simulink model "multiPhaseAFPM"  (R2022a)
settings: Solver=FixedStepAuto  StartTime=0.0  StopTime=T_end  FixedStep=T_sim  RelTol=1e-3
values from neighbouring files (symbols this model uses):
  fe = 0    [initializationScript.m]
  Id3_ref1 = 0    [initializationScript.m]
  Id3_ref2 = 0    [initializationScript.m]
  Id3_step = 0    [initializationScript.m]
  Id5_ref1 = 0    [initializationScript.m]
  Id5_ref2 = 0    [initializationScript.m]
  Id5_step = 0.0    (= 0)    [initializationScript.m]
  Id_ref1 = 0    [initializationScript.m]
  Id_ref2 = 0    [initializationScript.m]
  Id_step = 0    [initializationScript.m]
  Iq3_ref1 = 0    [initializationScript.m]
  Iq3_ref2 = 140    [initializationScript.m]
  Iq3_step = 0    [initializationScript.m]
  Iq5_ref1 = 0    [initializationScript.m]
  Iq5_ref2 = 0    [initializationScript.m]
  Iq5_step = 0    [initializationScript.m]
  Iq_ref1 = 0    [initializationScript.m]
  Iq_ref2 = 0    [initializationScript.m]
  Iq_step = 0    [initializationScript.m]
  L_ind1 = L1    (= 5e-05)    [initializationScript.m]
  L_ind2 = L1    (= 5e-05)    [initializationScript.m]
  L_ind3 = L1    (= 5e-05)    [initializationScript.m]
  L_ind4 = L1    (= 5e-05)    [initializationScript.m]
  L_ind5 = L1    (= 5e-05)    [initializationScript.m]
  L_ind6 = L1    (= 5e-05)    [initializationScript.m]
  L_ind7 = L1    (= 5e-05)    [initializationScript.m]
  PWM_INVERTER = 1    [initializationScript.m]
  R1 = R    (= 0.024)    [initializationScript.m]
  R2 = R    (= 0.024)    [initializationScript.m]
  R3 = R    (= 0.024)    [initializationScript.m]
  R4 = R    (= 0.024)    [initializationScript.m]
  R5 = R    (= 0.024)    [initializationScript.m]
  R6 = R    (= 0.024)    [initializationScript.m]
  R7 = R    (= 0.024)    [initializationScript.m]
  T_sim = Ts/200    (= 2e-07)    [initializationScript.m]
  Ts = 1/25000    (= 4e-05)    [initializationScript.m]
  Tsw = 1/Fsw    (= 1.66666666667e-05)    [initializationScript.m]
  VDC = 250    [initializationScript.m]
undefined symbols (not defined in the file or in its folder): R_ph
libraries: spsIdealSwitchLib x16, spsSeriesRLCBranchLib x14, spsCurrentMeasurementLib x7, simulink x1, spsDCVoltageSourceLib x1, spspowerguiLib x1
settings Model: Creator=anvar  LastModifiedBy=Nishanth
settings OptimizationCC: DefaultParameterBehavior=Inlined  EnhancedBackFolding=on  PassReuseOutputArgsAs=Individual arguments  ZeroExternalMemoryAtStartup=off  ZeroInternalMemoryAtStartup=off  OptimizeBlockOrder=speed  DifferentSizesBufferReuse=on  OptimizationCustomize=off  EfficientTunableParamExpr=on
settings DebuggingCC: ParameterTunabilityLossMsg=error  UnconnectedInputMsg=warning  UnconnectedOutputMsg=warning  UnconnectedLineMsg=warning
settings SFSimCC: MATLABDynamicMemAlloc=off
settings RTWCC: SystemTargetFile=ert.tlc  TemplateMakefile=ert_default_tmf  DLArmComputeVersion=19.05
settings CodeAppCC: ForceParamTrailComments=on  IgnoreCustomStorageClasses=off  OperatorAnnotations=on  SimulinkDataObjDesc=on  SFDataObjDesc=on  InsertBlockDesc=on
settings ERTTargetCC: TargetLangStandard=C99 (ISO)  GenerateSampleERTMain=on  InlinedParameterPlacement=NonHierarchical  ERTCustomFileTemplate=example_file_process.tlc

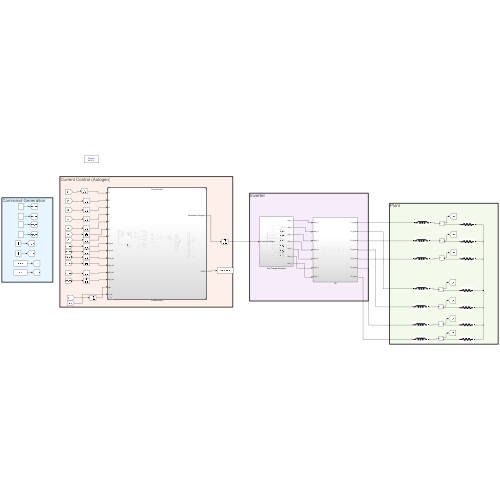
[thumbnail: Simulink's stored preview of the top-level diagram]
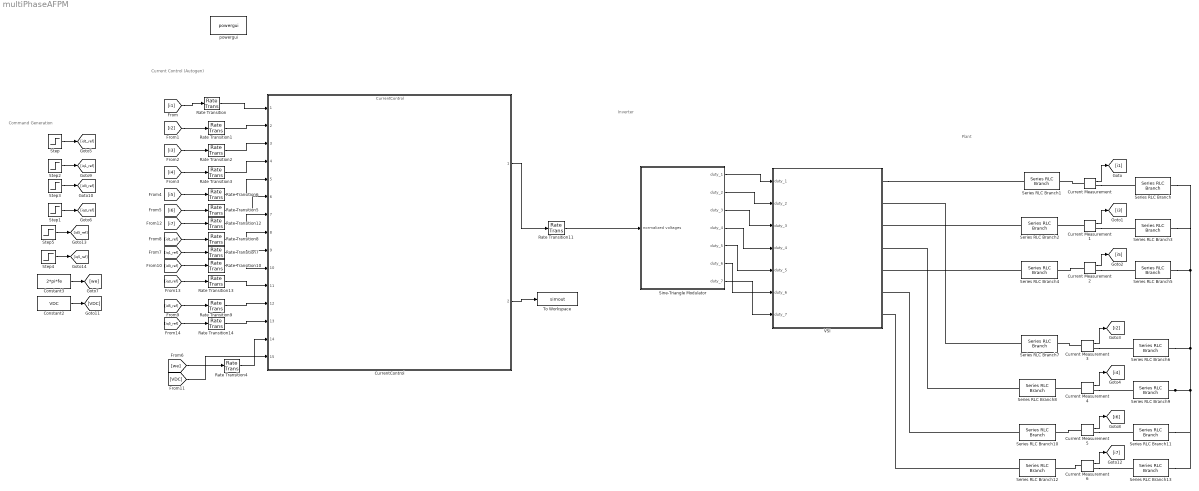
== system multiPhaseAFPM ==
  note: Plant
  note: Inverter
  note: Current Control (Autogen)
  note: Command Generation
  Constant2 : Constant  Value=VDC  SampleTime=Ts
  Constant3 : Constant  Value=2*pi*fe  SampleTime=Ts
  Current Measurement{,1..6} (7 alike) : spsCurrentMeasurementLib/Current Measurement  PhasorSimulation=off  OutputType=Complex  PSBequivalent=0
  CurrentControl : ModelReference  ModelNameDialog=CurrentControl  SimulationMode=Normal  ModelReferenceVersion=2.22
  Rate Transition{,1..10,12..14} (14 alike) : RateTransition  OutPortSampleTime=Ts
  Rate Transition11 : RateTransition  OutPortSampleTime=T_sim
  Series RLC Branch : spsSeriesRLCBranchLib/Series RLC Branch  LConnTagsString=__new0  RConnTagsString=__new0  BranchType=R  Resistance=R1  Inductance=1e-3  SetiL0=off  InitialCurrent=0  Capacitance=1e-6  Setx0=off  InitialVoltage=0  Measurements=None
  Series RLC Branch1 : spsSeriesRLCBranchLib/Series RLC Branch  LConnTagsString=__new0  RConnTagsString=__new0  BranchType=L  Resistance=R_ph  Inductance=L_ind1  SetiL0=off  InitialCurrent=0  Capacitance=1e-6  Setx0=off  InitialVoltage=0  Measurements=None
  Series RLC Branch10 : spsSeriesRLCBranchLib/Series RLC Branch  LConnTagsString=__new0  RConnTagsString=__new0  BranchType=L  Resistance=R_ph  Inductance=L_ind6  SetiL0=off  InitialCurrent=0  Capacitance=1e-6  Setx0=off  InitialVoltage=0  Measurements=None
  Series RLC Branch11 : spsSeriesRLCBranchLib/Series RLC Branch  LConnTagsString=__new0  RConnTagsString=__new0  BranchType=R  Resistance=R6  Inductance=1e-3  SetiL0=off  InitialCurrent=0  Capacitance=1e-6  Setx0=off  InitialVoltage=0  Measurements=None
  Series RLC Branch12 : spsSeriesRLCBranchLib/Series RLC Branch  LConnTagsString=__new0  RConnTagsString=__new0  BranchType=L  Resistance=R_ph  Inductance=L_ind7  SetiL0=off  InitialCurrent=0  Capacitance=1e-6  Setx0=off  InitialVoltage=0  Measurements=None
  Series RLC Branch13 : spsSeriesRLCBranchLib/Series RLC Branch  LConnTagsString=__new0  RConnTagsString=__new0  BranchType=R  Resistance=R7  Inductance=1e-3  SetiL0=off  InitialCurrent=0  Capacitance=1e-6  Setx0=off  InitialVoltage=0  Measurements=None
  Series RLC Branch2 : spsSeriesRLCBranchLib/Series RLC Branch  LConnTagsString=__new0  RConnTagsString=__new0  BranchType=L  Resistance=R_ph  Inductance=L_ind3  SetiL0=off  InitialCurrent=0  Capacitance=1e-6  Setx0=off  InitialVoltage=0  Measurements=None
  Series RLC Branch3 : spsSeriesRLCBranchLib/Series RLC Branch  LConnTagsString=__new0  RConnTagsString=__new0  BranchType=R  Resistance=R3  Inductance=1e-3  SetiL0=off  InitialCurrent=0  Capacitance=1e-6  Setx0=off  InitialVoltage=0  Measurements=None
  Series RLC Branch4 : spsSeriesRLCBranchLib/Series RLC Branch  LConnTagsString=__new0  RConnTagsString=__new0  BranchType=L  Resistance=R_ph  Inductance=L_ind5  SetiL0=off  InitialCurrent=0  Capacitance=1e-6  Setx0=off  InitialVoltage=0  Measurements=None
  Series RLC Branch5 : spsSeriesRLCBranchLib/Series RLC Branch  LConnTagsString=__new0  RConnTagsString=__new0  BranchType=R  Resistance=R5  Inductance=1e-3  SetiL0=off  InitialCurrent=0  Capacitance=1e-6  Setx0=off  InitialVoltage=0  Measurements=None
  Series RLC Branch6 : spsSeriesRLCBranchLib/Series RLC Branch  LConnTagsString=__new0  RConnTagsString=__new0  BranchType=R  Resistance=R2  Inductance=1e-3  SetiL0=off  InitialCurrent=0  Capacitance=1e-6  Setx0=off  InitialVoltage=0  Measurements=None
  Series RLC Branch7 : spsSeriesRLCBranchLib/Series RLC Branch  LConnTagsString=__new0  RConnTagsString=__new0  BranchType=L  Resistance=R_ph  Inductance=L_ind2  SetiL0=off  InitialCurrent=0  Capacitance=1e-6  Setx0=off  InitialVoltage=0  Measurements=None
  Series RLC Branch8 : spsSeriesRLCBranchLib/Series RLC Branch  LConnTagsString=__new0  RConnTagsString=__new0  BranchType=L  Resistance=R_ph  Inductance=L_ind4  SetiL0=off  InitialCurrent=0  Capacitance=1e-6  Setx0=off  InitialVoltage=0  Measurements=None
  Series RLC Branch9 : spsSeriesRLCBranchLib/Series RLC Branch  LConnTagsString=__new0  RConnTagsString=__new0  BranchType=R  Resistance=R4  Inductance=1e-3  SetiL0=off  InitialCurrent=0  Capacitance=1e-6  Setx0=off  InitialVoltage=0  Measurements=None
  Sine-Triangle Modulator : Subsystem
  Step : Step  Time=Id_step  Before=Id_ref1  After=Id_ref2  SampleTime=Ts  mask(DiscretizedSource){}
      mask init:
      | %zoh
  Step1 : Step  Time=Iq3_step  Before=Iq3_ref1  After=Iq3_ref2  SampleTime=Ts  mask(DiscretizedSource){}
      mask init:
      | %zoh
  Step2 : Step  Time=Iq_step  Before=Iq_ref1  After=Iq_ref2  SampleTime=Ts  mask(DiscretizedSource){}
      mask init:
      | %zoh
  Step3 : Step  Time=Id3_step  Before=Id3_ref1  After=Id3_ref2  SampleTime=Ts  mask(DiscretizedSource){}
      mask init:
      | %zoh
  Step4 : Step  Time=Iq5_step  Before=Iq5_ref1  After=Iq5_ref2  SampleTime=Ts  mask(DiscretizedSource){}
      mask init:
      | %zoh
  Step5 : Step  Time=Id5_step  Before=Id5_ref1  After=Id5_ref2  SampleTime=Ts  mask(DiscretizedSource){}
      mask init:
      | %zoh
  To Workspace : ToWorkspace  VariableName=simout  SaveFormat=Timeseries  SampleTime=-1
  VSI : Subsystem
  powergui : spspowerguiLib/powergui  Priority=1  SimulationMode=Discrete  SampleTime=T_sim  frequency=60  Iterations=50  frequencyindice=0  Pbase=100e6  ErrMax=1e-4  UnitsV=kV  UnitsW=MW  buscounter=0  FunctionMessages=off  echomessages=off  EnableUseOfTLC=off  CurrentSourceSwitches=off  DisableSnubberDevices=off  DisableRonSwitches=off  DisableVfSwitches=off  DisplayEquations=off  AutomaticDiscreteSolvers=off  SolverType=Tustin/Backward Euler (TBE)  Interpol=off  ExternalGateDelay=off  methode=off  Ts=100  x0status=blocks  SPID=on  SwTol=0  HookPort=off  NonlinearTolerance=1e-4  nMaxIteration=100  ContinueOnMaxIteration=off  RestoreLinks=warning  ResistiveCurrentMeasurement=off  Frange=[0:2:500]  Ylog=off  Xlog=on  ShowGrid=off  save=off  variable=ZData  structure=0  ZoomFFT=off  StartTime=0.0  cycles=1  DisplayStyle=1  fundamental=60  FreqAxis=off  MaxFrequency=1000  frequencyindicesteady=1  RmsSteady=1  display=off
  wires:
  [i6] -> Rate Transition5/1
  [we] -> Rate Transition4/1
  [i1] -> Rate Transition/1
  [i2] -> Rate Transition1/1
  [i3] -> Rate Transition2/1
  [i4] -> Rate Transition3/1
  [i5] -> Rate Transition6/1
  [iq1_ref] -> Rate Transition7/1
  [id1_ref] -> Rate Transition8/1
  [id5_ref] -> Rate Transition9/1
  [id3_ref] -> Rate Transition10/1
  CurrentControl/1 -> Rate Transition11/1
  Rate Transition11/1 -> Sine-Triangle Modulator/1(normalized voltages)
  Sine-Triangle Modulator/1(duty_1) -> VSI/1(duty_1)
  Sine-Triangle Modulator/2(duty_2) -> VSI/2(duty_2)
  Sine-Triangle Modulator/3(duty_3) -> VSI/3(duty_3)
  Sine-Triangle Modulator/4(duty_4) -> VSI/4(duty_4)
  Sine-Triangle Modulator/5(duty_5) -> VSI/5(duty_5)
  Sine-Triangle Modulator/6(duty_6) -> VSI/6(duty_6)
  Constant3/1 -> [we]
  Step/1 -> [id1_ref]
  Step1/1 -> [iq3_ref]
  Current Measurement1/1 -> [i3]
  Current Measurement/1 -> [i1]
  Current Measurement2/1 -> [i5]
  Rate Transition2/1 -> CurrentControl/3
  Rate Transition3/1 -> CurrentControl/4
  Rate Transition1/1 -> CurrentControl/2
  Rate Transition/1 -> CurrentControl/1
  Current Measurement5/1 -> [i6]
  Current Measurement3/1 -> [i2]
  Current Measurement4/1 -> [i4]
  Step3/1 -> [id3_ref]
  Step2/1 -> [iq1_ref]
  Constant2/1 -> [VDC]
  Current Measurement6/1 -> [i7]
  [i7] -> Rate Transition12/1
  [iq3_ref] -> Rate Transition13/1
  [iq5_ref] -> Rate Transition14/1
  Sine-Triangle Modulator/7(duty_7) -> VSI/7(duty_7)
  Step5/1 -> [id5_ref]
  Step4/1 -> [iq5_ref]
  CurrentControl/2 -> To Workspace/1
  Rate Transition9/1 -> CurrentControl/12
  Rate Transition14/1 -> CurrentControl/13
  Rate Transition4/1 -> CurrentControl/14
  [VDC] -> CurrentControl/15
  Rate Transition10/1 -> CurrentControl/10
  Rate Transition13/1 -> CurrentControl/11
  Rate Transition7/1 -> CurrentControl/9
  Rate Transition8/1 -> CurrentControl/8
  Rate Transition12/1 -> CurrentControl/7
  Rate Transition5/1 -> CurrentControl/6
  Rate Transition6/1 -> CurrentControl/5
  connections:
  Series RLC Branch2/LConn1 -- VSI/RConn3
  Current Measurement2/RConn1 -- Series RLC Branch5/LConn1
  Current Measurement/LConn1 -- Series RLC Branch1/RConn1
  Current Measurement1/LConn1 -- Series RLC Branch2/RConn1
  Current Measurement/RConn1 -- Series RLC Branch/LConn1
  Current Measurement1/RConn1 -- Series RLC Branch3/LConn1
  Series RLC Branch4/LConn1 -- VSI/RConn5
  Current Measurement2/LConn1 -- Series RLC Branch4/RConn1
  Series RLC Branch9/RConn1 -- Series RLC Branch5/RConn1 -- Series RLC Branch3/RConn1 -- Series RLC Branch/RConn1 -- Series RLC Branch6/RConn1 -- Series RLC Branch13/RConn1 -- Series RLC Branch11/RConn1
  Current Measurement5/LConn1 -- Series RLC Branch10/RConn1
  Series RLC Branch10/LConn1 -- VSI/RConn6
  Current Measurement4/RConn1 -- Series RLC Branch9/LConn1
  Current Measurement4/LConn1 -- Series RLC Branch8/RConn1
  Series RLC Branch7/LConn1 -- VSI/RConn2
  Current Measurement5/RConn1 -- Series RLC Branch11/LConn1
  Current Measurement3/RConn1 -- Series RLC Branch6/LConn1
  Series RLC Branch8/LConn1 -- VSI/RConn4
  Current Measurement3/LConn1 -- Series RLC Branch7/RConn1
  VSI/RConn1 -- Series RLC Branch1/LConn1
  Current Measurement6/LConn1 -- Series RLC Branch12/RConn1
  Current Measurement6/RConn1 -- Series RLC Branch13/LConn1
  Series RLC Branch12/LConn1 -- VSI/RConn7

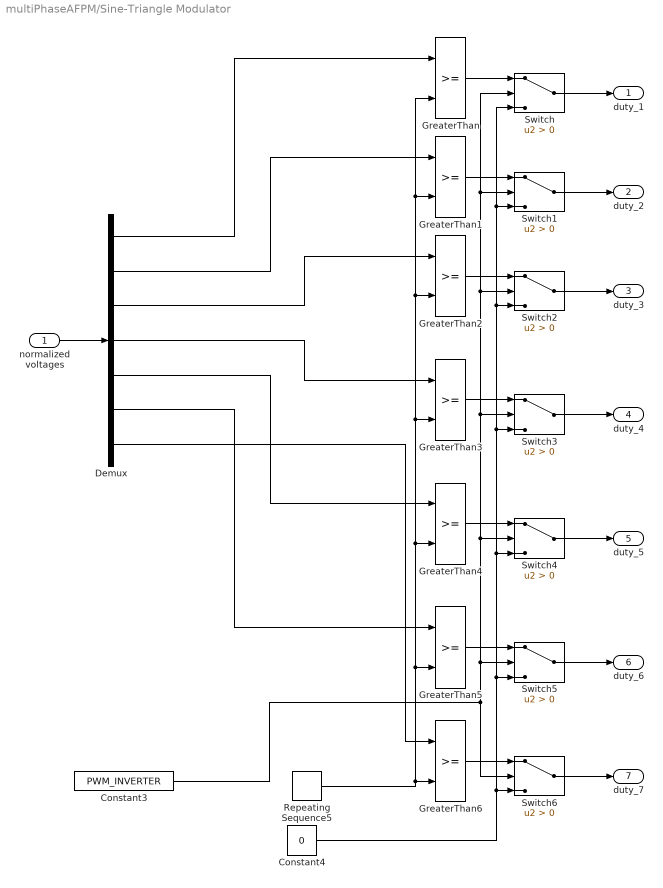
== system multiPhaseAFPM/Sine-Triangle Modulator ==
  normalized voltages : Inport
  Constant3 : Constant  Value=PWM_INVERTER
  Constant4 : Constant  Value=0
  Demux : Demux  Outputs=7
  GreaterThan{,1..6} (7 alike) : RelationalOperator  OutDataTypeStr=boolean  RndMeth=Simplest  InputSameDT=off
  Repeating Sequence5 : simulink/Sources/Repeating Sequence  rep_seq_t=[0 Tsw/2 Tsw]  rep_seq_y=[-1 1 -1]
  Switch{,1..6} (7 alike) : Switch  Criteria=u2 > Threshold  SaturateOnIntegerOverflow=off  InputSameDT=off
  duty_1 : Outport
  duty_2 : Outport  Port=2
  duty_3 : Outport  Port=3
  duty_4 : Outport  Port=4
  duty_5 : Outport  Port=5
  duty_6 : Outport  Port=6
  duty_7 : Outport  Port=7
  wires:
  GreaterThan2/1 -> Switch2/1
  GreaterThan1/1 -> Switch1/1
  GreaterThan/1 -> Switch/1
  Repeating Sequence5/1 -> GreaterThan6/2, GreaterThan/2, GreaterThan1/2, GreaterThan2/2, GreaterThan3/2, GreaterThan4/2, GreaterThan5/2
  Switch2/1 -> duty_3/1
  Switch1/1 -> duty_2/1
  Switch/1 -> duty_1/1
  normalized voltages/1 -> Demux/1
  Switch3/1 -> duty_4/1
  GreaterThan3/1 -> Switch3/1
  GreaterThan4/1 -> Switch4/1
  Switch4/1 -> duty_5/1
  Switch5/1 -> duty_6/1
  GreaterThan5/1 -> Switch5/1
  Demux/1 -> GreaterThan/1
  Demux/2 -> GreaterThan1/1
  Demux/3 -> GreaterThan2/1
  Demux/4 -> GreaterThan3/1
  Demux/5 -> GreaterThan4/1
  Demux/6 -> GreaterThan5/1
  Constant3/1 -> Switch6/2, Switch/2, Switch1/2, Switch2/2, Switch3/2, Switch4/2, Switch5/2
  Constant4/1 -> Switch6/3, Switch3/3, Switch/3, Switch1/3, Switch2/3, Switch4/3, Switch5/3
  GreaterThan6/1 -> Switch6/1
  Switch6/1 -> duty_7/1
  Demux/7 -> GreaterThan6/1

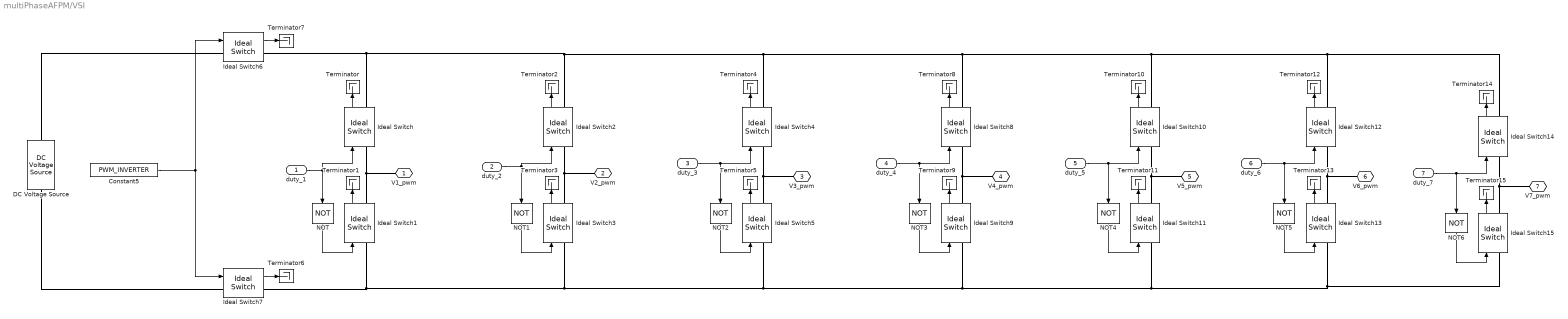
== system multiPhaseAFPM/VSI ==
  duty_1 : Inport
  duty_2 : Inport  Port=2
  duty_3 : Inport  Port=3
  duty_4 : Inport  Port=4
  duty_5 : Inport  Port=5
  duty_6 : Inport  Port=6
  duty_7 : Inport  Port=7
  Constant5 : Constant  Value=PWM_INVERTER
  DC Voltage Source : spsDCVoltageSourceLib/DC Voltage Source  Amplitude=VDC  Measurements=None
  Ideal Switch{,1..15} (16 alike) : spsIdealSwitchLib/Ideal Switch  Ron=0.001  Lon=0  IC=0  Rs=1e5  Cs=inf  Measurements=on
  NOT{,1..6} (7 alike) : Logic  Operator=NOT  IconShape=distinctive  AllPortsSameDT=off  OutDataTypeStr=boolean
  Terminator{,1..15} (16 alike) : Terminator
  V1_pwm : PMIOPort  Tag=PMCPort  Side=Right
  V2_pwm : PMIOPort  Tag=PMCPort  Port=2  Side=Right
  V3_pwm : PMIOPort  Tag=PMCPort  Port=3  Side=Right
  V4_pwm : PMIOPort  Tag=PMCPort  Port=4  Side=Right
  V5_pwm : PMIOPort  Tag=PMCPort  Port=5  Side=Right
  V6_pwm : PMIOPort  Tag=PMCPort  Port=6  Side=Right
  V7_pwm : PMIOPort  Tag=PMCPort  Port=7  Side=Right
  wires:
  duty_2/1 -> Ideal Switch2/1, NOT1/1
  Ideal Switch4/1 -> Terminator4/1
  Ideal Switch/1 -> Terminator/1
  Ideal Switch2/1 -> Terminator2/1
  Ideal Switch1/1 -> Terminator1/1
  NOT/1 -> Ideal Switch1/1
  Ideal Switch5/1 -> Terminator5/1
  Ideal Switch3/1 -> Terminator3/1
  NOT2/1 -> Ideal Switch5/1
  duty_3/1 -> NOT2/1, Ideal Switch4/1
  Ideal Switch6/1 -> Terminator7/1
  duty_1/1 -> Ideal Switch/1, NOT/1
  Constant5/1 -> Ideal Switch6/1, Ideal Switch7/1
  NOT1/1 -> Ideal Switch3/1
  Ideal Switch7/1 -> Terminator6/1
  duty_4/1 -> Ideal Switch8/1, NOT3/1
  NOT3/1 -> Ideal Switch9/1
  Ideal Switch9/1 -> Terminator9/1
  Ideal Switch8/1 -> Terminator8/1
  Ideal Switch10/1 -> Terminator10/1
  Ideal Switch11/1 -> Terminator11/1
  NOT4/1 -> Ideal Switch11/1
  duty_5/1 -> NOT4/1, Ideal Switch10/1
  duty_6/1 -> Ideal Switch12/1, NOT5/1
  NOT5/1 -> Ideal Switch13/1
  Ideal Switch13/1 -> Terminator13/1
  Ideal Switch12/1 -> Terminator12/1
  Ideal Switch15/1 -> Terminator15/1
  NOT6/1 -> Ideal Switch15/1
  duty_7/1 -> Ideal Switch14/1, NOT6/1
  Ideal Switch14/1 -> Terminator14/1
  connections:
  DC Voltage Source/LConn1 -- Ideal Switch7/LConn1
  Ideal Switch2/RConn1 -- Ideal Switch14/RConn1 -- Ideal Switch12/RConn1 -- Ideal Switch10/RConn1 -- Ideal Switch8/RConn1 -- Ideal Switch4/RConn1 -- Ideal Switch6/RConn1 -- Ideal Switch/RConn1
  Ideal Switch/LConn1 -- Ideal Switch1/RConn1 -- V1_pwm/RConn1
  Ideal Switch4/LConn1 -- Ideal Switch5/RConn1 -- V3_pwm/RConn1
  Ideal Switch2/LConn1 -- Ideal Switch3/RConn1 -- V2_pwm/RConn1
  Ideal Switch3/LConn1 -- Ideal Switch15/LConn1 -- Ideal Switch13/LConn1 -- Ideal Switch11/LConn1 -- Ideal Switch9/LConn1 -- Ideal Switch5/LConn1 -- Ideal Switch7/RConn1 -- Ideal Switch1/LConn1
  DC Voltage Source/RConn1 -- Ideal Switch6/LConn1
  Ideal Switch8/LConn1 -- V4_pwm/RConn1 -- Ideal Switch9/RConn1
  V5_pwm/RConn1 -- Ideal Switch10/LConn1 -- Ideal Switch11/RConn1
  Ideal Switch12/LConn1 -- V6_pwm/RConn1 -- Ideal Switch13/RConn1
  Ideal Switch15/RConn1 -- Ideal Switch14/LConn1 -- V7_pwm/RConn1
